simulink model "rtwdemo_advsc"  (Simulink 7.6)
settings: Solver=FixedStepDiscrete  StartTime=0.0  StopTime=10.0  FixedStep=1  RelTol=1e-3
PostLoadFcn:
  | open_system('rtwdemo_advsc/Auto');
values from neighbouring files (symbols this model uses):
  K1 = 3    [rtwdemo_cgv_init.m]    (also in rtwdemo_dow_data.m)
undefined symbols (not defined in the file or in its folder): LOWER, T1Break, T1Data, T2Data, UPPER
libraries: rtwdemowidgets x3
Description:
  | Data Dictionary Driven Modeling Using Simulink(R) Data Objects
settings Model: Creator=The MathWorks Inc.  CovMetricSettings=d  ExtModeAutoUpdateStatusClock=off
settings MATStruct: SampleTime=1  Offset=0  Priority=[20.0]
settings DataIOCC: SaveOutput=off  SaveTime=off  SignalLoggingName=sigsOut
settings OptimizationCC: InlineParams=on  InlineInvariantSignals=on  PassReuseOutputArgsAs=Individual arguments  StateBitsets=on  DataBitsets=on  UseTempVars=on  ZeroExternalMemoryAtStartup=off  ZeroInternalMemoryAtStartup=off  NoFixptDivByZeroProtection=on  EfficientFloat2IntCast=on  EfficientMapNaN2IntZero=off  OptimizeModelRefInitCode=on  LifeSpan=1
settings DebuggingCC: CheckExecutionContextPreStartOutputMsg=on  CheckExecutionContextRuntimeOutputMsg=on  SolverPrmCheckMsg=none  ParameterUnderflowMsg=error  ParameterPrecisionLossMsg=none  StrictBusMsg=ErrorOnBusTreatedAsVector
settings HardwareCC: ProdIntDivRoundTo=Zero  ProdEndianess=LittleEndian  ProdHWDeviceType=Generic->32-bit Embedded Processor  TargetHWDeviceType=Generic->32-bit Embedded Processor
settings SFSimCC: SimParseCustomCode=off
settings RTWCC: SystemTargetFile=ert.tlc  TLCOptions=-p0  TemplateMakefile=ert_default_tmf  Description=Real-Time Workshop Embedded Coder (no auto configuration)  GenerateReport=on  RTWVerbose=off  ProcessScript=ert_make_rtw_hook  IncludeHyperlinkInReport=on  LaunchReport=on
settings CodeAppCC: ForceParamTrailComments=on  IgnoreCustomStorageClasses=off  IgnoreTestpoints=on
settings ERTTargetCC: TargetFcnLib=ansi_tfl_tmw.mat  MultiwordLength=2048  GenerateSampleERTMain=on  SupportNonFinite=off  InlinedParameterPlacement=NonHierarchical  ERTCustomFileTemplate=example_file_process.tlc  ConvertIfToSwitch=off

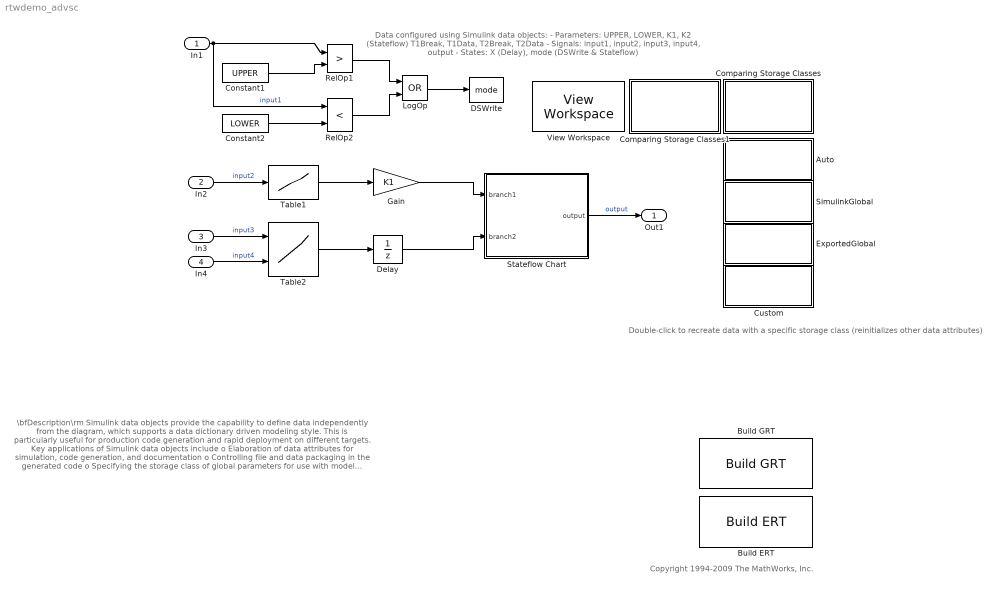
== system rtwdemo_advsc ==
  note: Data configured using Simulink data objects:
      | - Parameters: UPPER, LOWER, K1, K2 (Stateflow)
      |                            T1Break, T1Data, T2Break, T2Data
      | - Signals: input1, input2, input3, input4, output
      | - States: X (Delay), mode (DSWrite & Stateflow)
  note: \bfDescription\rm
      | Simulink data objects provide the capability to define data independently from the
      | diagram, which supports a data dictionary driven modeling style.  This is particularly
      | useful for production code generation and rapid deployment on different targets.
      |
      | Key applications of Simulink data objects include
      |
      | o Elaboration of data attributes for simulation, code generation, and documentation
      | o Controlling file and data packaging in the generated code
      | o Specifying the storage class of global parameters for use with model reference
      | o Generating ASAP2 and other calibration data files
      |
      | \bfInstructions\rm
      | 1. Open the Model Explorer to view and modify the attributes of workspace variables.
      |      For example, change the definition of MYTYPE and then update the diagram.
      | 2. Double-click the boxes on the right to recreate the data or generate code.
      |
      | \bfNotes\rm
      | o MYTYPE is a user-defined data type object.  Preserving this data type name in
      |    the generated code requires a Real-Time Workshop Embedded Coder license.
      | o Real-Time Workshop supports built-in storage classes.  Custom storage
      |    classes require a Real-Time Workshop Embedded Coder license.
  note: Double-click to recreate data
      | with a specific storage class
      | (reinitializes other data attributes)
  note: Copyright 1994-2009 The MathWorks, Inc.
  In1 : Inport  OutDataTypeStr=MYTYPE  PortDimensions=1  SampleTime=1
  In2 : Inport  Port=2  OutDataTypeStr=MYTYPE  PortDimensions=1  SampleTime=1
  In3 : Inport  Port=3  OutDataTypeStr=MYTYPE  PortDimensions=1  SampleTime=1
  In4 : Inport  Port=4  OutDataTypeStr=MYTYPE  PortDimensions=1  SampleTime=1
  Auto : Subsystem  mask(Advanced data packaging - create data){StorageClass=Auto, DataInitFcn=rtwdemo_advsc_data}
      mask help: OpenFcn creates data with the specified storage class for data packaging demo.
      mask init:
      | dispStr = 'Initialize data with\nStorageClass: ';
      | dispStr = [dispStr, StorageClass];
      settings: OpenFcn=feval(get_param(gcb, 'DataInitFcn'), get_param(gcb, 'StorageClass'));
      mask StyleString: popup(Auto|SimulinkGlobal|ExportedGlobal|Custom),edit
      mask Display: disp([StorageClass, '\nStorage Class']);
  Build ERT : rtwdemowidgets/Build ERT  SystemSampleTime=-1  attrib_overrides={}
  Build GRT : rtwdemowidgets/Build GRT  SystemSampleTime=-1  attrib_overrides={}
  Comparing Storage Classes : Subsystem
      mask Display: disp(['Compare the\noptions ..', '.\n(double-click)']);
  Comparing Storage Classes1 : Subsystem
      settings: OpenFcn=edit rtwdemo_advsc_data
      mask Display: disp(['View M-File\nData Source\n(double-click)']);
  Constant1 : Constant  Value=UPPER  OutDataTypeStr=Inherit: Inherit via back propagation
  Constant2 : Constant  Value=LOWER  OutDataTypeStr=Inherit: Inherit via back propagation
  Custom : Subsystem  mask(Advanced data packaging - create data){StorageClass=Custom, DataInitFcn=rtwdemo_advsc_data}
      mask help: OpenFcn creates data with the specified storage class for data packaging demo.
      mask init:
      | dispStr = 'Initialize data with\nStorageClass: ';
      | dispStr = [dispStr, StorageClass];
      settings: OpenFcn=feval(get_param(gcb, 'DataInitFcn'), get_param(gcb, 'StorageClass'));
      mask StyleString: popup(Auto|SimulinkGlobal|ExportedGlobal|Custom),edit
      mask Display: disp([StorageClass, '\nStorage Class']);
  DSWrite : DataStoreWrite  DataStoreName=mode
  Delay : UnitDelay  SampleTime=-1  StateIdentifier=X  StateMustResolveToSignalObject=on
  ExportedGlobal : Subsystem  mask(Advanced data packaging - create data){StorageClass=ExportedGlobal, DataInitFcn=rtwdemo_advsc_data}
      mask help: OpenFcn creates data with the specified storage class for data packaging demo.
      mask init:
      | dispStr = 'Initialize data with\nStorageClass: ';
      | dispStr = [dispStr, StorageClass];
      settings: OpenFcn=feval(get_param(gcb, 'DataInitFcn'), get_param(gcb, 'StorageClass'));
      mask StyleString: popup(Auto|SimulinkGlobal|ExportedGlobal|Custom),edit
      mask Display: disp([StorageClass, '\nStorage Class']);
  Gain : Gain  Gain=K1  SaturateOnIntegerOverflow=on  OutDataTypeStr=Inherit: Same as input  ParamDataTypeStr=Inherit: Same as input
  LogOp : Logic  Operator=OR
  RelOp1 : RelationalOperator  Operator=>  InputSameDT=on
  RelOp2 : RelationalOperator  Operator=<  InputSameDT=on
  SimulinkGlobal : Subsystem  mask(Advanced data packaging - create data){StorageClass=SimulinkGlobal, DataInitFcn=rtwdemo_advsc_data}
      mask help: OpenFcn creates data with the specified storage class for data packaging demo.
      mask init:
      | dispStr = 'Initialize data with\nStorageClass: ';
      | dispStr = [dispStr, StorageClass];
      settings: OpenFcn=feval(get_param(gcb, 'DataInitFcn'), get_param(gcb, 'StorageClass'));
      mask StyleString: popup(Auto|SimulinkGlobal|ExportedGlobal|Custom),edit
      mask Display: disp([StorageClass, '\nStorage Class']);
  Stateflow Chart : Stateflow chart  TreatAsAtomicUnit=on
  Table1 : Lookup  InputValues=T1Break  Table=T1Data  LookUpMeth=Interpolation-Use End Values  SaturateOnIntegerOverflow=on
  Table2 : Lookup2D  RowIndex=T2Break  ColumnIndex=T2Break  Table=T2Data  LookUpMeth=Interpolation-Use End Values  InputSameDT=on
  View Workspace : rtwdemowidgets/View Workspace  SystemSampleTime=-1
  Out1 : Outport
  wires:
  RelOp1/1 -> LogOp/1
  RelOp2/1 -> LogOp/2
  Constant2/1 -> RelOp2/2
  In2/1 -> Table1/1  "input2"
  Gain/1 -> Stateflow Chart/1(branch1)
  Table1/1 -> Gain/1
  Table2/1 -> Delay/1
  Constant1/1 -> RelOp1/2
  In1/1 -> RelOp2/1, RelOp1/1  "input1"
  In3/1 -> Table2/1  "input3"
  In4/1 -> Table2/2  "input4"
  Stateflow Chart/1(output) -> Out1/1  "output"
  Delay/1 -> Stateflow Chart/2(branch2)
  LogOp/1 -> DSWrite/1

== system rtwdemo_advsc/Auto ==

== system rtwdemo_advsc/Comparing Storage Classes ==
  note: NOTE: All descriptions assume that the inline parameters and signal storage reuse optimizations are ON.
  note: 1. Auto storage class:
      |
      | Motivation:
      | - Maximize efficiency of the generated code
      |
      | Behavior:
      | - Parameters are inlined and intermediate signals are eliminated
      | - All states and root-level I/O are members of persistent data structures
      |
      | Advantages:
      | - Optimized code generation
      | - Default behavior when optimizations enabled (easy to use)
      |
      | Disadvantages:
      | - Parameters and signals do not appear as variables in the generated code
  note: 2. SimulinkGlobal storage class:
      |
      | Motivation:
      | - Provide visibility (persistence) for selected data
      |
      | Behavior:
      | - Select parameters and signals are members of persistent data structures
      | - All states and root-level I/O are members of persistent data structures
      |
      | Advantages:
      | - Only increase memory usage for data of interest
      | - Provides visibility to data without limiting modeling flexibility and code efficiency
      |
      | Disadvantages:
      | - Minimal control over variable names
  note: 3. Unstructured storage classes (e.g., ExportedGlobal):
      |
      | Motivation:
      | - Interface to global data in hand-written (legacy) code
      |
      | Behavior:
      | - Select parameters and signals are global, unstructured variables
      | - Select states and root-level I/O are global, unstructured variables
      |
      | Advantages:
      | - Data names are preserved in the generated code
      |
      | Disadvantages:
      | - Imposes certain modeling restrictions
      | - Disables certain code optimizations
  note: 4. Custom storage classes (CSCs):
      |
      | Motivation:
      | - Generate custom (user-defined) data packaging to conform with
      |     virtually any legacy data packaging and development process
      |
      | Behavior:
      | - Representation determined by custom storage class definitions
      |
      | Advantages:
      | - Full control over location, packaging and format of data
      | - Control over comments and pragmas (compiler directives)
      |
      | Disadvantages:
      | - Imposes certain modeling restrictions
      | - Disables certain code optimizations

== system rtwdemo_advsc/Comparing Storage Classes1 ==
  note: 4. Custom storage classes (CSCs):
      |
      | Motivation:
      | - Generate custom (user-defined) data packaging to conform with
      |     virtually any legacy data packaging and development process
      |
      | Behavior:
      | - Representation determined by custom storage class definitions
      |
      | Advantages:
      | - Full control over location, packaging and format of data
      | - Control over comments and pragmas (compiler directives)
      |
      | Disadvantages:
      | - Imposes certain modeling restrictions
      | - Disables certain code optimizations
  note: 3. Unstructured storage classes (e.g., ExportedGlobal):
      |
      | Motivation:
      | - Interface to global data in hand-written (legacy) code
      |
      | Behavior:
      | - Select parameters and signals are global, unstructured variables
      | - Select states and root-level I/O are global, unstructured variables
      |
      | Advantages:
      | - Data names are preserved in the generated code
      |
      | Disadvantages:
      | - Imposes certain modeling restrictions
      | - Disables certain code optimizations
  note: 2. SimulinkGlobal storage class:
      |
      | Motivation:
      | - Provide visibility (persistence) for selected data
      |
      | Behavior:
      | - Select parameters and signals are members of persistent data structures
      | - All states and root-level I/O are members of persistent data structures
      |
      | Advantages:
      | - Only increase memory usage for data of interest
      | - Provides visibility to data without limiting modeling flexibility and code efficiency
      |
      | Disadvantages:
      | - Minimal control over variable names
  note: 1. Auto storage class:
      |
      | Motivation:
      | - Maximize efficiency of the generated code
      |
      | Behavior:
      | - Parameters are inlined and intermediate signals are eliminated
      | - All states and root-level I/O are members of persistent data structures
      |
      | Advantages:
      | - Optimized code generation
      | - Default behavior when optimizations enabled (easy to use)
      |
      | Disadvantages:
      | - Parameters and signals do not appear as variables in the generated code
  note: NOTE: All descriptions assume that the inline parameters and signal storage reuse optimizations are ON.

== system rtwdemo_advsc/Custom ==

== system rtwdemo_advsc/ExportedGlobal ==

== system rtwdemo_advsc/SimulinkGlobal ==

== stateflow chart Stateflow Chart ==
  note: This chart implements an if-else condition, based
      | on the value of data store memory "mode".
      | The result is multiplied by parameter "K2".
      |
      | Using a Simulink switch (or if-action) and gain block,
      |     results in virtually identical code.
  (junction 7) -> (junction 4) : {output = branch1;}
  (junction 4) -> (junction 6) : {output *= K2;}
  (junction 5) -> (junction 4) [order 2] : {output = branch2;}
  (default) -> (junction 5)
  (junction 5) -> (junction 7) [order 1] : [mode]
  data: branch1 input double; mode data_store_memory double; branch2 input double; output output type(branch1) size=size(branch1); K2 parameter double
